simulink model "three_phase_full_controled"  (R2018a)
settings: Solver=VariableStepAuto  StartTime=0.0  StopTime=0.1  RelTol=1e-3
undefined symbols (not defined in the file): D1, lagging, pulse
libraries: powerlib x14, powerlib_meascontrol x2
settings Model: Creator=31295  LastModifiedBy=31295

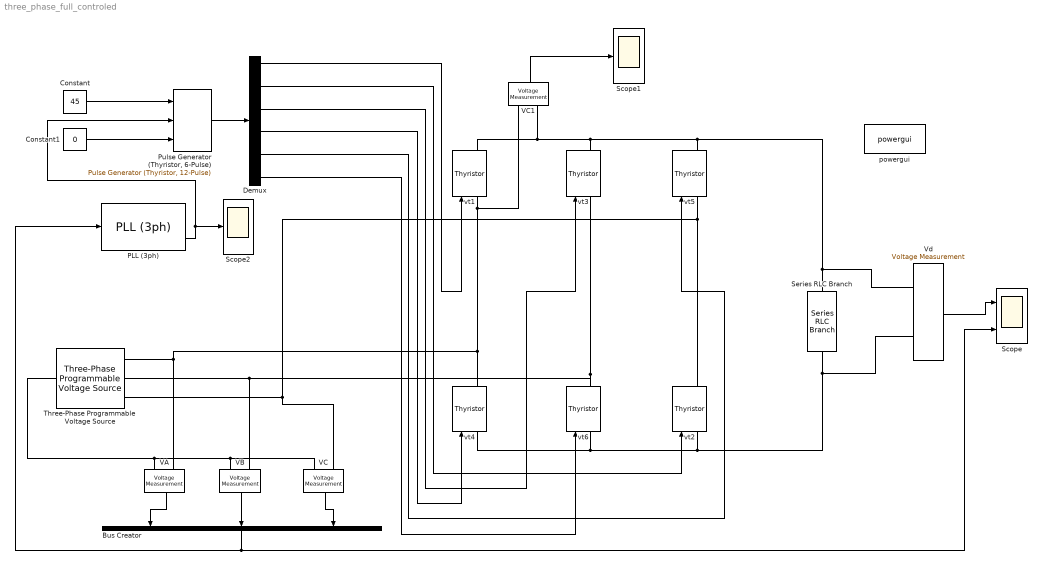
== system three_phase_full_controled ==
  " VC" : powerlib/Measurements/Voltage Measurement  PhasorSimulation=off  OutputType=Complex  PSBequivalent=0
  " VC1" : powerlib/Measurements/Voltage Measurement  PhasorSimulation=off  OutputType=Complex  PSBequivalent=0
  Bus Creator : BusCreator  Inputs=3
  Constant : Constant  Value=45
  Constant1 : Constant  Value=0
  Demux : Demux  Outputs=6
  PLL (3ph) : powerlib_meascontrol/PLL/PLL (3ph)  Fmin=45  Par_Init=[0, 50]  ParK=[90, 1600, 1]  TcD=1e-4  MaxRateChangeFreq=12  FilterCutOffFreq=25  Ts=0  AGC=on
  "Pulse Generator (Thyristor, 6-Pulse)" : powerlib_meascontrol/Pulse & Signal Generators/Pulse Generator (Thyristor, 12-Pulse)  GenType=6-pulse  Delta=D1 (lagging)  pwidth=10  Double_Pulse=on  Ts=0
      settings: SourceProductName=Simscape Power Systems  SourceProductBaseCode=PS
  Scope : Scope  NumInputPorts=2
  Scope1 : Scope
  Scope2 : Scope
  Series RLC Branch : powerlib/Elements/Series RLC Branch  LConnTagsString=__new0  RConnTagsString=__new0  BranchType=R  Resistance=10  Inductance=1e-3  SetiL0=off  InitialCurrent=0  Capacitance=1e-6  Setx0=off  InitialVoltage=0  Measurements=None
  Three-Phase Programmable Voltage Source : powerlib/Electrical Sources/Three-Phase Programmable Voltage Source  PositiveSequence="[220  0 50]"  VariationEntity=None  VariationType=Table of time-amplitude pairs  VariationTypeAlt=Step  VariationStep=0.5  VariationRate=10  VariationMagnitude=0.3  VariationFrequency=2  VariationTiming=[1 2]  VariationPhaseA=off  Amplitudes=[1 0.8 1.2 1.0]  TimeValues=[0 0.1 0.15 0.2]  HarmonicGeneration=off  HarmonicA=[3 0.2 -25 0]  HarmonicB=[2 0.15 35 2]  Timing="[0.05  3]"  BusType=swing  Pref=0  Qref=0  Qmin=-inf  Qmax=inf
  VA : powerlib/Measurements/Voltage Measurement  PhasorSimulation=off  OutputType=Complex  PSBequivalent=0
  VB : powerlib/Measurements/Voltage Measurement  PhasorSimulation=off  OutputType=Complex  PSBequivalent=0
  Vd : powerlib/Measurements/Voltage Measurement  PhasorSimulation=off  OutputType=Complex  PSBequivalent=0
  powergui : powerlib/powergui  Priority=1  SimulationMode=Continuous  SampleTime=50e-6  frequency=60  Iterations=50  frequencyindice=50  Pbase=100e6  ErrMax=1e-4  UnitsV=kV  UnitsW=MW  buscounter=0  FunctionMessages=off  echomessages=off  EnableUseOfTLC=off  CurrentSourceSwitches=off  DisableSnubberDevices=off  DisableRonSwitches=off  DisableVfSwitches=off  DisplayEquations=off  SolverType=Tustin/Backward Euler (TBE)  Interpol=off  ExternalGateDelay=off  methode=off  Ts=100  x0status=blocks  SPID=on  SwTol=0  HookPort=off  RestoreLinks=warning  ResistiveCurrentMeasurement=off  Frange=[0:2:500]  Ylog=off  Xlog=on  ShowGrid=off  save=off  variable=ZData  structure=0  ZoomFFT=off  StartTime=0.0  cycles=1  DisplayStyle=1  fundamental=60  FreqAxis=off  MaxFrequency=1000  frequencyindicesteady=1  RmsSteady=1  display=off
  vt{1..3,5..6} (5 alike) : powerlib/Power Electronics/Thyristor  Ron=0.001  Lon=0  Vf=0.8  IC=0  Rs=500  Cs=250e-9  Measurements=on
  "vt4 " : powerlib/Power Electronics/Thyristor  Ron=0.001  Lon=0  Vf=0.8  IC=0  Rs=500  Cs=250e-9  Measurements=on
  wires:
  Constant/1 -> "Pulse Generator (Thyristor, 6-Pulse)"/1
  Constant1/1 -> "Pulse Generator (Thyristor, 6-Pulse)"/3
  "Pulse Generator (Thyristor, 6-Pulse)"/1 -> Demux/1
  Demux/1 -> vt1/1
  Demux/2 -> vt2/1
  Demux/3 -> vt3/1
  Demux/4 -> "vt4 "/1
  Demux/5 -> vt5/1
  Demux/6 -> vt6/1
  Vd/1 -> Scope/1
  VA/1 -> Bus Creator/1
  VB/1 -> Bus Creator/2
  " VC"/1 -> Bus Creator/3
  Bus Creator/1 -> PLL (3ph)/1, Scope/2
  PLL (3ph)/2 -> "Pulse Generator (Thyristor, 6-Pulse)"/2, Scope2/1
  " VC1"/1 -> Scope1/1
  connections:
  vt1/RConn1 -- " VC1"/LConn2 -- Vd/LConn1 -- Series RLC Branch/LConn1 -- vt5/RConn1 -- vt3/RConn1
  vt6/LConn1 -- Vd/LConn2 -- Series RLC Branch/RConn1 -- vt2/LConn1 -- "vt4 "/LConn1
  vt3/LConn1 -- Three-Phase Programmable Voltage Source/RConn2 -- VB/LConn1 -- vt6/RConn1
  vt5/LConn1 -- " VC"/LConn1 -- Three-Phase Programmable Voltage Source/RConn3 -- vt2/RConn1
  vt1/LConn1 -- " VC1"/LConn1 -- VA/LConn1 -- Three-Phase Programmable Voltage Source/RConn1 -- "vt4 "/RConn1
  VA/LConn2 -- Three-Phase Programmable Voltage Source/LConn1 -- " VC"/LConn2 -- VB/LConn2
